simulink model "NMPCLib"  (R2018a)
settings: Solver=VariableStepAuto  StartTime=0.0  StopTime=4000  RelTol=1e-3  EnableMultiTasking=on
values from neighbouring files (symbols this model uses):
  Cai = 3.3*0.001    (= 0.0033)    [Data.m]
  Cair = 0.3    [Data.m]    (also in go.m = 0.4; go_params.m = 0.4)
  Cap = 45*3600    (= 162000)    [Data.m]
  Cb = 14000*3.56    (= 49840)    [Data.m]
  Cc = 43667.5*0.896    (= 39126.08)    [Data.m]
  Cd = 0.4*0.996    (= 0.3984)    [Data.m]
  Ci = 5*0.001    (= 0.005)    [Data.m]
  Cl = 560*0.896    (= 501.76)    [Data.m]
  Co = 3000*0.921    (= 2763)    [Data.m]
  dU0 = 0*ones(Usize,1)    [go.m]
  g = 9.8    [Data.m]    (also in go.m; go_params.m)
  Ja = 0.7282    [Data.m]
  Jb = 0.7282    [Data.m]
  Kb = 9.6    [Data.m]
  Kre_a = 0.10    (= 0.1)    [Data.m]
  Kre_b = 0.12    [Data.m]
  Ktr = 4.4    [Data.m]
  M = 288    [Data.m]    (also in go.m; go_params.m)
  Miur0 = 0.01    [Data.m]    (also in go.m; go_params.m)
  Np = ceil(45/6.650)    [Data.m]
  Ns = ceil(72/12.6)    [Data.m]
  pair = 1.25    [Data.m]    (also in go.m = 0.9643; go_params.m = 0.9643)
  Qrd = as*(GD*cos(ang)+Gd)    [Data.m]
  Raic = 1/(Aaic*h_air)    (= 406.940119575)    [Data.m]
  Rail = 1/(Alai*h_air)    (= 951.594301092)    [Data.m]
  Rba = 1/(Aba*k_litio)    (= 0.0922236978014)    [Data.m]
  Rbi = 1/(Abi*k_litio)    (= 0.0277596414787)    [Data.m]
  Rbo = 1/(Abo*k_litio)    (= 0.0277596414787)    [Data.m]
  Rca = 1/(Aca*k_alum)    (= 0.0351745602272)    [Data.m]
  Rcai = 1/(Aaic*k_alum)    (= 0.0505515676491)    [Data.m]
  Rdl = 1/(Adl*(k_alum*km_Crem))    (= 0.0199076286033)    [Data.m]
  Rib = 1/(Abi*h_air)    (= 321.584769745)    [Data.m]
  Rio = 1/(Aio*h_air)    (= 898.634076204)    [Data.m]
  Rlai = 1/(Alai*k_alum)    (= 0.118210472185)    [Data.m]
  Rlc = 1/(Alc*k_alum)    (= 0.115635579282)    [Data.m]
  Roa = 1/(Aoa*k_alum)    (= 0.029420140793)    [Data.m]
  Rob = 1/(Abo*k_alum)    (= 0.0399484186019)    [Data.m]
  Roi = 1/(Aio*k_alum)    (= 0.111631562261)    [Data.m]
  Rwr = 0.3302    [Data.m]    (also in go.m = 0.58; go_params.m = 0.58)
  Surf = 0.94243    [Data.m]    (also in go.m; go_params.m)
  Tai0 = 25    [Data.m]
  Tb0 = 25    [Data.m]
  Tc0 = 25    [Data.m]
  Td0 = 25    [Data.m]
  Ti0 = 25    [Data.m]
  Tl0 = 25    [Data.m]
  To0 = 25    [Data.m]
  U0 = 0*ones(Usize,1)    [go.m]
  Udc = 72    [Data.m]
libraries: simulink x6
settings Model: Creator=stajeddi  LastModifiedBy=yesid
settings DataIOCC: LimitDataPoints=on
settings OptimizationCC: LifeSpan=inf
settings DebuggingCC: AllowSymbolicDim=off  SFUnexpectedBacktrackingDiag=warning  SFNoUnconditionalDefaultTransitionDiag=warning  SFExecutionAtInitializationDiag=none
settings ModelReferenceCC: PropagateSignalLabelsOutOfModel=off
settings CodeAppCC: StateflowObjectComments=on
settings GRTTargetCC: TargetLangStandard=C89/C90 (ANSI)
settings ConfigComp: CovMetricSettings=dw  CovHtmlReporting=on  CovSaveCumulativeToWorkspaceVar=on  CovSaveSingleToWorkspaceVar=on  CovExternalEMLEnable=off

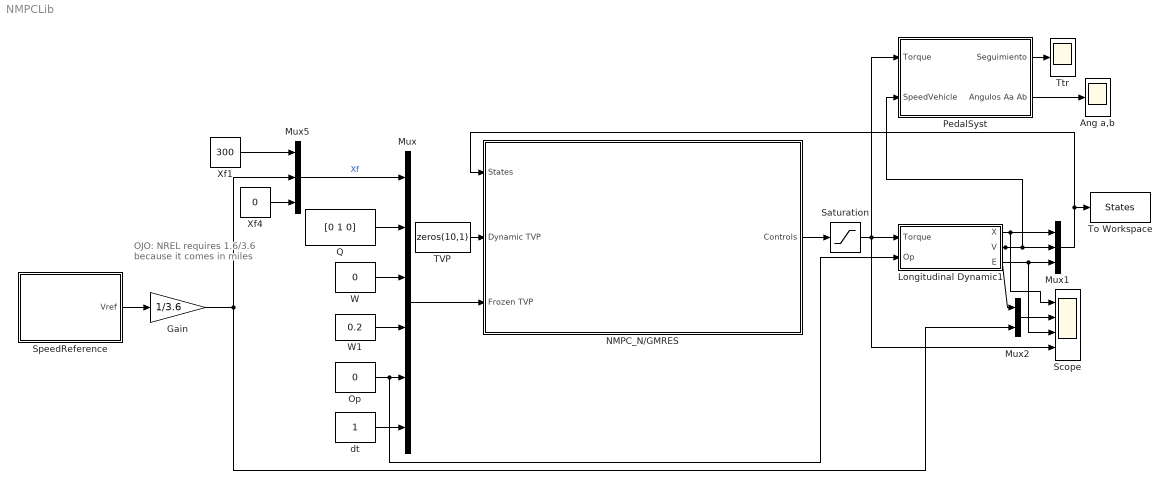
== system NMPCLib ==
  note: OJO: NREL requires
      | 1.6/3.6 because it
      | comes in miles
  Ang a,b : Scope
  Gain : Gain  Gain=1/3.6
  Longitudinal Dynamic1 : Subsystem
  Mux : Mux  Inputs=6
  Mux1 : Mux  Inputs=3
  Mux2 : Mux  Inputs=2
  Mux5 : Mux  Inputs=3
  NMPC_N/GMRES : Subsystem
  Op : Constant  Value=0
  PedalSyst : Subsystem
  Q : Constant  Value=[0 1 0]
  Saturation : Saturate  UpperLimit=220  LowerLimit=-220
  Scope : Scope  NumInputPorts=4
  "SpeedReference " : Subsystem
  TVP : Constant  Value=zeros(10,1)
  To Workspace : ToWorkspace  VariableName=States  SaveFormat=Timeseries  SampleTime=-1
  "Ttr " : Scope
  W : Constant  Value=0
  W1 : Constant  Value=0.2
  Xf1 : Constant  Value=300
  Xf4 : Constant  Value=0
  dt : Constant
  wires:
  Mux/1 -> NMPC_N/GMRES/3(Frozen TVP)
  Q/1 -> Mux/2
  W/1 -> Mux/3
  Mux5/1 -> Mux/1  "Xf"
  TVP/1 -> NMPC_N/GMRES/2(Dynamic TVP)
  Longitudinal Dynamic1/1(X) -> Scope/1, Mux1/1
  Longitudinal Dynamic1/2(V) -> Mux2/1, PedalSyst/2(SpeedVehicle), Mux1/2
  Xf1/1 -> Mux5/1
  Op/1 -> Longitudinal Dynamic1/2("Op "), Mux/5
  Mux2/1 -> Scope/2
  W1/1 -> Mux/4
  dt/1 -> Mux/6
  Xf4/1 -> Mux5/3
  Longitudinal Dynamic1/3(E) -> Scope/3, Mux1/3
  "SpeedReference "/1(Vref) -> Gain/1
  PedalSyst/1(Seguimiento) -> "Ttr "/1
  PedalSyst/2(Angulos Aa Ab) -> Ang a,b/1
  NMPC_N/GMRES/1(Controls) -> Saturation/1
  Saturation/1 -> PedalSyst/1(Torque), Scope/4, Longitudinal Dynamic1/1(Torque)
  Gain/1 -> Mux2/2, Mux5/2
  Mux1/1 -> To Workspace/1, NMPC_N/GMRES/1(States)

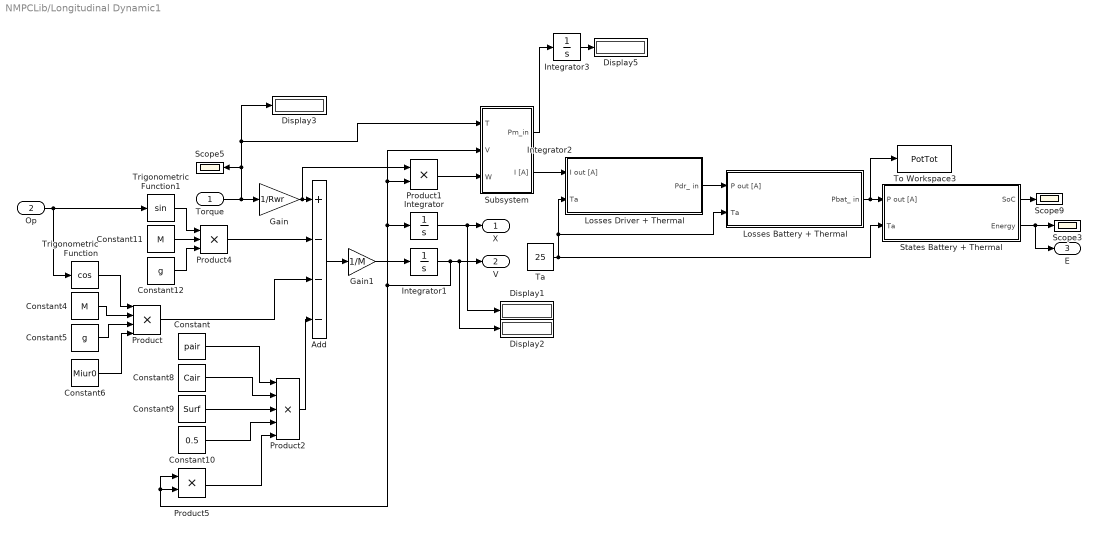
== system NMPCLib/Longitudinal Dynamic1 ==
  Torque : Inport
  "Op " : Inport  Port=2
  Add : Sum  Inputs=+---
  Constant : Constant  Value=pair
  Constant10 : Constant  Value=0.5
  Constant11 : Constant  Value=M
  Constant12 : Constant  Value=g
  Constant4 : Constant  Value=M
  Constant5 : Constant  Value=g
  Constant6 : Constant  Value=Miur0
  Constant8 : Constant  Value=Cair
  Constant9 : Constant  Value=Surf
  Display{1..3,5} (4 alike) : Display
  Gain : Gain  Gain=1/Rwr
  Gain1 : Gain  Gain=1/M
  Integrator{,1..3} (4 alike) : Integrator
  Losses Battery + Thermal : Subsystem
  Losses Driver + Thermal : Subsystem
  Product : Product  Inputs=4
  Product1 : Product
  Product2 : Product  Inputs=5
  Product4 : Product  Inputs=3
  Product5 : Product
  Scope3 : Scope
  Scope5 : Scope
  Scope9 : Scope
  States Battery + Thermal : Subsystem
  Subsystem : Subsystem
  Ta : Constant  Value=25
  To Workspace3 : ToWorkspace  VariableName=PotTot  SaveFormat=Timeseries  SampleTime=-1
  Trigonometric Function : Trigonometry  Operator=cos
  Trigonometric Function1 : Trigonometry
  X : Outport
  V : Outport  Port=2
  E : Outport  Port=3
  wires:
  Integrator/1 -> X/1, Display1/1
  Product2/1 -> Add/4
  Product5/1 -> Product2/5
  Constant10/1 -> Product2/4
  Constant8/1 -> Product2/2
  Constant/1 -> Product2/1
  Constant9/1 -> Product2/3
  Product/1 -> Add/3
  Constant6/1 -> Product/4
  Trigonometric Function/1 -> Product/1
  Constant5/1 -> Product/3
  Constant4/1 -> Product/2
  Add/1 -> Gain1/1
  "Op "/1 -> Trigonometric Function1/1, Trigonometric Function/1
  Product4/1 -> Add/2
  Gain/1 -> Product1/1, Add/1
  Constant12/1 -> Product4/3
  Trigonometric Function1/1 -> Product4/1
  Constant11/1 -> Product4/2
  Gain1/1 -> Integrator1/1
  Integrator1/1 -> V/1, Display2/1, Product1/2, Subsystem/2(V), Integrator/1, Product5/1, Product5/2
  Product1/1 -> Subsystem/3(W)
  Subsystem/1("Pm_in ") -> Integrator3/1
  Integrator3/1 -> Display5/1
  Subsystem/2(I [A]) -> Losses Driver + Thermal/1(I out [A])
  Losses Battery + Thermal/1(Pbat_ in) -> To Workspace3/1, States Battery + Thermal/1(P out [A])
  Ta/1 -> States Battery + Thermal/2(Ta), Losses Battery + Thermal/2(Ta), Losses Driver + Thermal/2(Ta)
  States Battery + Thermal/1(SoC) -> Scope9/1
  States Battery + Thermal/2(Energy) -> E/1, Scope3/1
  Torque/1 -> Gain/1, Scope5/1, Subsystem/1(T), Display3/1
  Losses Driver + Thermal/1(Pdr_ in) -> Losses Battery + Thermal/1(P out [A])

== system NMPCLib/NMPC_N//GMRES ==
  States : Inport
  Dynamic TVP : Inport  Port=2
  Frozen TVP : Inport  Port=3
  Solver : MATLAB Function  TreatAsAtomicUnit=on
  U0 : UnitDelay  InitialCondition=U0  SampleTime=-1
  dU0 : UnitDelay  InitialCondition=dU0  SampleTime=-1
  Controls : Outport
  wires:
  States/1 -> Solver/3(x0)
  Frozen TVP/1 -> Solver/5(TVP_f)
  Solver/3(Control) -> Controls/1
  Solver/2(U) -> U0/1
  U0/1 -> Solver/2(U0)
  Solver/1(dU) -> dU0/1
  dU0/1 -> Solver/1(dU0)
  Dynamic TVP/1 -> Solver/4(TVP)

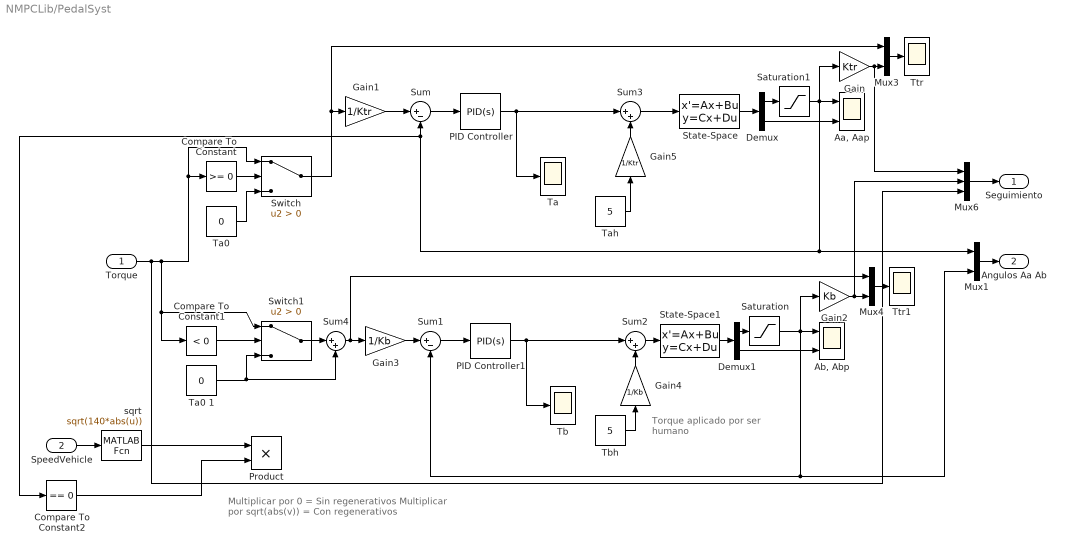
== system NMPCLib/PedalSyst ==
  note: Torque aplicado
      | por ser humano
  note: Multiplicar por 0                 = Sin regenerativos
      | Multiplicar por sqrt(abs(v)) = Con regenerativos
  Torque : Inport
  SpeedVehicle : Inport  Port=2
  "Aa, Aap" : Scope  NumInputPorts=2
  "Ab, Abp" : Scope  NumInputPorts=2
  Compare To Constant : simulink/Logic and Bit Operations/Compare To Constant  relop=>=  const=0  OutDataTypeStr=boolean
  Compare To Constant1 : simulink/Logic and Bit Operations/Compare To Constant  relop=<  const=0  OutDataTypeStr=boolean
  Compare To Constant2 : simulink/Logic and Bit Operations/Compare To Constant  relop===  const=0  OutDataTypeStr=boolean
  Demux : Demux  Outputs=2
  Demux1 : Demux  Outputs=2
  Gain : Gain  Gain=Ktr
  Gain1 : Gain  Gain=1/Ktr
  Gain2 : Gain  Gain=Kb
  Gain3 : Gain  Gain=1/Kb
  Gain4 : Gain  Gain=1/Kb
  Gain5 : Gain  Gain=1/Ktr
  Mux1 : Mux  Inputs=2
  Mux3 : Mux  Inputs=2
  Mux4 : Mux  Inputs=2
  Mux6 : Mux  Inputs=3
  PID Controller : simulink/Continuous/PID Controller  Controller=PID  TimeDomain=Continuous-time  SampleTime=-1  IntegratorMethod=Forward Euler  FilterMethod=Forward Euler  Form=Parallel  UseFilter=on  ControllerParametersSource=internal  P=1.77054619183816  I=0.294850673068489  D=2.09654617749741  N=11.2597730875944  InitialConditionSource=internal  InitialConditionForIntegrator=0  InitialConditionForFilter=0  ExternalReset=none  LimitOutput=off  UpperSaturationLimit=inf  LowerSaturationLimit=-inf  LinearizeAsGain=on  AntiWindupMode=none  Kb=1  TrackingMode=off  Kt=1  PParamMin=[]  PParamMax=[]  IParamMin=[]  IParamMax=[]  DParamMin=[]  DParamMax=[]  NParamMin=[]  NParamMax=[]  KbParamMin=[]  KbParamMax=[]  KtParamMin=[]  KtParamMax=[]  POutMin=[]  POutMax=[]  IOutMin=[]  IOutMax=[]  DOutMin=[]  DOutMax=[]  NOutMin=[]  NOutMax=[]  KbOutMin=[]  KbOutMax=[]  KtOutMin=[]  KtOutMax=[]  IntegratorOutMin=[]  IntegratorOutMax=[]  FilterOutMin=[]  FilterOutMax=[]  SumOutMin=[]  SumOutMax=[]  SumI1OutMin=[]  SumI1OutMax=[]  SumI2OutMin=[]  SumI2OutMax=[]  SumI3OutMin=[]  SumI3OutMax=[]  SumDOutMin=[]  SumDOutMax=[]  SaturationOutMin=[]  SaturationOutMax=[]  IntegratorContinuousStateAttributes=''  IntegratorStateMustResolveToSignalObject=off  IntegratorRTWStateStorageClass=Auto  FilterContinuousStateAttributes=''  FilterStateMustResolveToSignalObject=off  FilterRTWStateStorageClass=Auto  DifferentiatorICPrevScaledInput=0  DifferentiatorOutMin=[]  DifferentiatorOutMax=[]  FilterDiffOutCoefMin=[]  FilterDiffOutCoefMax=[]  SumDenOutMin=[]  SumDenOutMax=[]  SumNumOutMin=[]  SumNumOutMax=[]  ReciprocalOutMin=[]  ReciprocalOutMax=[]  DivideOutMin=[]  DivideOutMax=[]  TunerSelectOption=Transfer Function Based (PID Tuner App)
  PID Controller1 : simulink/Continuous/PID Controller  Controller=PID  TimeDomain=Continuous-time  SampleTime=-1  IntegratorMethod=Forward Euler  FilterMethod=Forward Euler  Form=Parallel  UseFilter=on  ControllerParametersSource=internal  P=1.6606981855622  I=0.298062139202914  D=2.01708670293522  N=30.9007600848216  InitialConditionSource=internal  InitialConditionForIntegrator=0  InitialConditionForFilter=0  ExternalReset=none  LimitOutput=off  UpperSaturationLimit=inf  LowerSaturationLimit=-inf  LinearizeAsGain=on  AntiWindupMode=none  Kb=1  TrackingMode=off  Kt=1  PParamMin=[]  PParamMax=[]  IParamMin=[]  IParamMax=[]  DParamMin=[]  DParamMax=[]  NParamMin=[]  NParamMax=[]  KbParamMin=[]  KbParamMax=[]  KtParamMin=[]  KtParamMax=[]  POutMin=[]  POutMax=[]  IOutMin=[]  IOutMax=[]  DOutMin=[]  DOutMax=[]  NOutMin=[]  NOutMax=[]  KbOutMin=[]  KbOutMax=[]  KtOutMin=[]  KtOutMax=[]  IntegratorOutMin=[]  IntegratorOutMax=[]  FilterOutMin=[]  FilterOutMax=[]  SumOutMin=[]  SumOutMax=[]  SumI1OutMin=[]  SumI1OutMax=[]  SumI2OutMin=[]  SumI2OutMax=[]  SumI3OutMin=[]  SumI3OutMax=[]  SumDOutMin=[]  SumDOutMax=[]  SaturationOutMin=[]  SaturationOutMax=[]  IntegratorContinuousStateAttributes=''  IntegratorStateMustResolveToSignalObject=off  IntegratorRTWStateStorageClass=Auto  FilterContinuousStateAttributes=''  FilterStateMustResolveToSignalObject=off  FilterRTWStateStorageClass=Auto  DifferentiatorICPrevScaledInput=0  DifferentiatorOutMin=[]  DifferentiatorOutMax=[]  FilterDiffOutCoefMin=[]  FilterDiffOutCoefMax=[]  SumDenOutMin=[]  SumDenOutMax=[]  SumNumOutMin=[]  SumNumOutMax=[]  ReciprocalOutMin=[]  ReciprocalOutMax=[]  DivideOutMin=[]  DivideOutMax=[]  TunerSelectOption=Transfer Function Based (PID Tuner App)
  Product : Product
  Saturation : Saturate  UpperLimit=0  LowerLimit=-50
  Saturation1 : Saturate  UpperLimit=50  LowerLimit=0
  State-Space : StateSpace  A=[0 1; -Kre_a/Ja 0]  B=[0; 1/Ja]  C=[1 0; 0 1]  D=[0; 0]  InitialCondition=[0 0]
  State-Space1 : StateSpace  A=[0 1; -Kre_b/Jb 0]  B=[0; 1/Jb]  C=[1 0; 0 1]  D=[0; 0]  InitialCondition=[0 0]
  Sum : Sum  Inputs=|+-
  Sum1 : Sum  Inputs=|+-
  Sum2 : Sum  Inputs=|++
  Sum3 : Sum  Inputs=|++
  Sum4 : Sum  Inputs=|++
  Switch : Switch  Criteria=u2 > Threshold
  Switch1 : Switch  Criteria=u2 > Threshold
  Ta : Scope
  "Ta0 " : Constant  Value=0
  Ta0 1 : Constant  Value=0
  Tah : Constant  Value=5
  Tb : Scope
  "Tbh " : Constant  Value=5
  Ttr : Scope
  Ttr1 : Scope
  sqrt : MATLABFcn  MATLABFcn=sqrt(140*abs(u))
  Seguimiento : Outport
  Angulos Aa Ab : Outport  Port=2
  wires:
  "Ta0 "/1 -> Switch/3
  Gain2/1 -> Mux6/2, Mux4/2
  Gain5/1 -> Sum3/2
  Torque/1 -> Switch/1, Compare To Constant/1, Switch1/1, Compare To Constant1/1, Mux6/3
  PID Controller1/1 -> Sum2/1, Tb/1
  Switch/1 -> Mux3/1, Gain1/1
  Gain/1 -> Mux6/1, Mux3/2
  Gain1/1 -> Sum/1
  Ta0 1/1 -> Sum4/2, Switch1/3
  Tah/1 -> Gain5/1
  Compare To Constant/1 -> Switch/2
  PID Controller/1 -> Sum3/1, Ta/1
  Sum/1 -> PID Controller/1
  Sum3/1 -> State-Space/1
  State-Space/1 -> Demux/1
  Compare To Constant1/1 -> Switch1/2
  Mux6/1 -> Seguimiento/1
  Mux4/1 -> Ttr1/1
  Sum2/1 -> State-Space1/1
  Demux/2 -> "Aa, Aap"/2
  "Tbh "/1 -> Gain4/1
  State-Space1/1 -> Demux1/1
  Mux3/1 -> Ttr/1
  Sum1/1 -> PID Controller1/1
  Gain4/1 -> Sum2/2
  Gain3/1 -> Sum1/1
  Demux1/2 -> "Ab, Abp"/2
  Mux1/1 -> Angulos Aa Ab/1
  Demux1/1 -> Saturation/1
  Saturation/1 -> Mux1/2, Sum1/2, Gain2/1, "Ab, Abp"/1
  Demux/1 -> Saturation1/1
  Saturation1/1 -> Sum/2, Compare To Constant2/1, Mux1/1, Gain/1, "Aa, Aap"/1
  Switch1/1 -> Sum4/1
  Sum4/1 -> Mux4/1, Gain3/1
  SpeedVehicle/1 -> sqrt/1
  sqrt/1 -> Product/1
  Compare To Constant2/1 -> Product/2

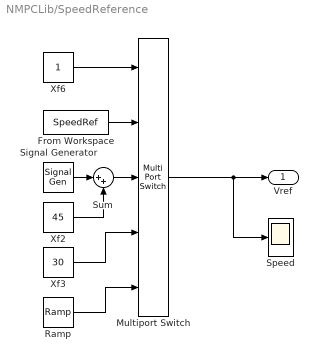
== system NMPCLib/SpeedReference  ==
  From Workspace : FromWorkspace  VariableName=SpeedRef  SampleTime=0
  Multiport Switch : MultiPortSwitch  Inputs=4
  Ramp : simulink/Sources/Ramp  slope=0.03  start=0  InitialOutput=0
  Signal Generator : SignalGenerator  Units=rad/sec
  "Speed " : Scope
  Sum : Sum  Inputs=|++
  Xf2 : Constant  Value=45
  Xf3 : Constant  Value=30
  Xf6 : Constant
  Vref : Outport
  wires:
  Signal Generator/1 -> Sum/1
  From Workspace/1 -> Multiport Switch/2
  Xf6/1 -> Multiport Switch/1
  Ramp/1 -> Multiport Switch/5
  Xf3/1 -> Multiport Switch/4
  Xf2/1 -> Sum/2
  Sum/1 -> Multiport Switch/3
  Multiport Switch/1 -> "Speed "/1, Vref/1

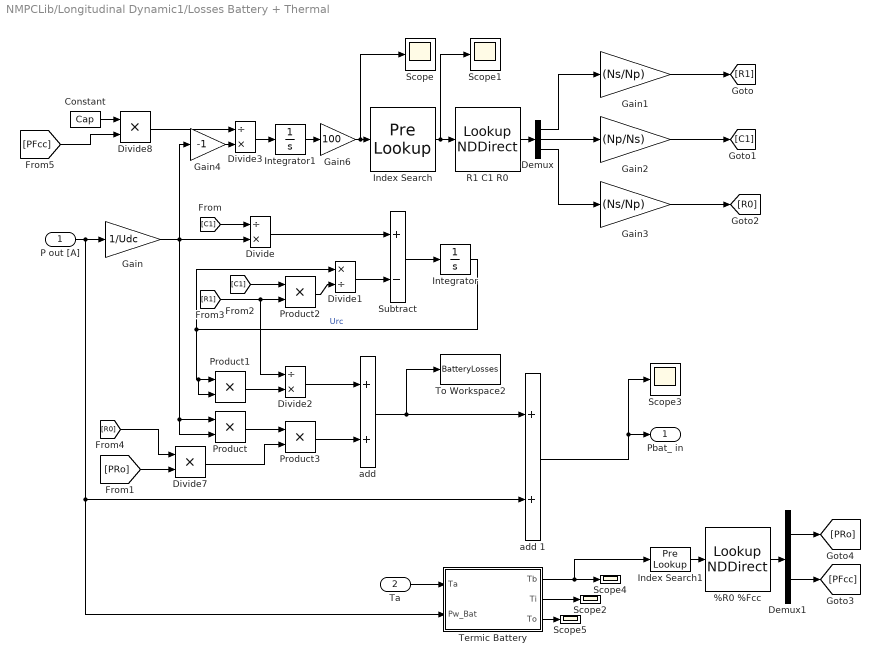
== system NMPCLib/Longitudinal Dynamic1/Losses Battery + Thermal ==
  P out [A] : Inport
  Ta : Inport  Port=2
  "%R0 %Fcc " : LookupNDDirect  InputsSelectThisObjectFromTable=Vector  Table=|
      | [7.33  0.71;
      | 4.97  0.75;
      | 3.58  0.78;
      | 2.69  0.82;
      | 2.07  0.86;
      | 1.63  0.89;
      | 1.30  0.93;
      | 1.14  0.97;
      | 1.00  1.00;
      | 0.91  1.04;
      | 0.84  1.07;
      | 0.77  1.09;]'
  Constant : Constant  Value=Cap
  Demux : Demux  Outputs=3
  Demux1 : Demux  Outputs=2
  Divide : Product  Inputs=/*
  Divide1 : Product  Inputs=*/
  Divide2 : Product  Inputs=/*
  Divide3 : Product  Inputs=/*
  Divide7 : Product  Inputs=**
  Divide8 : Product  Inputs=**
  Gain : Gain  Gain=1/Udc
  Gain1 : Gain  Gain=(Ns/Np)
  Gain2 : Gain  Gain=(Np/Ns)
  Gain3 : Gain  Gain=(Ns/Np)
  Gain4 : Gain  Gain=-1
  Gain6 : Gain  Gain=100
  Index Search : PreLookup  BreakpointsData=|  OutputSelection=Index only
      | [2.273
      | 4.545
      | 6.818
      | 9.091
      | 11.364
      | 13.636
      | 15.909
      | 18.182
      | 20.455
      | 22.727
      | 25.000
      | 27.273
      | 29.545
      | 31.818
      | 34.091
      | 36.364
      | 38.636
      | 40.909
      | 43.182
      | 45.455
      | 47.727
      | 50.000
      | 52.273
      | 54.545
      | 56.818
      | 59.091
      | 61.364
      | 63.636
      | 65.909
      | 68.182
      | 70.455
      | 72.727
      | 75.000
      | 77.273
      | 79.545
      | 81.818
      | 84.091
      | 86.364
      | 88.636
      | 90.909
      | 93.182
      | 95.455
      | 97.727
      | 100.000]
  Index Search1 : PreLookup  BreakpointsData="[-15 -10 -5 0  5 10  15 20 25 30 35 40]"  OutputSelection=Index only
  Integrator : Integrator
  Integrator1 : Integrator  InitialCondition=1
  Product{,1..3} (4 alike) : Product
  "R1 C1 R0 " : LookupNDDirect  InputsSelectThisObjectFromTable=Vector  Table=|
      | [0.046  1443.329 0.260;
      | 0.163	383.931	0.260;
      | 0.264	202.535	0.262;
      | 0.301	109.504	0.263;
      | 0.303	99.992	0.260;
      | 0.303	107.088	0.263;
      | 0.298	126.400	0.262;
      | 0.307	131.885	0.263;
      | 0.303	119.317	0.260;
      | 0.304	125.895	0.260;
      | 0.309	113.359	0.260;
      | 0.307	107.787	0.260;
      | 0.306	117.780	0.262;
      | 0.313	104.457	0.262;
      | 0.310	100.585	0.258;
      | 0.304	136.742	0.260;
      | 0.310	126.376	0.262;
      | 0.313	126.403	0.260;
      | 0.309	110.120	0.257;
      | 0.315	114.389	0.258;
      | 0.314	98.257	0.260;
      | 0.314	95.395	0.260;
      | 0.319	88.712	0.257;
      | 0.320	77.705	0.258;
      | 0.319	78.111	0.258;
      | 0.325	69.286	0.260;
      | 0.322	90.719	0.257;
      | 0.331	91.019	0.262;
      | 0.313	100.060	0.257;
      | 0.317	108.165	0.262;
      | 0.313	130.331	0.258;
      | 0.304	128.624	0.255;
      | 0.300	139.477	0.253;
      | 0.303	143.003	0.255;
      | 0.313	129.373	0.258;
      | 0.318	129.417	0.258;
      | 0.313	107.012	0.255;
      | 0.326	96.506	0.260;
      | 0.328	83.578	0.258;
      | 0.337	95.942	0.263;
      | 0.344	86.032	0.267;
      | 0.351	59.468	0.270;
      | 0.318	101.474	0.255;
      | 0.283	133.248	0.127;]'
  Scope{,1..5} (6 alike) : Scope
  Subtract : Sum  Inputs=+-
  "Termic Battery " : Subsystem
  To Workspace2 : ToWorkspace  VariableName=BatteryLosses  SaveFormat=Timeseries  SampleTime=-1
  "add " : Sum
  add 1 : Sum
  Pbat_ in : Outport
  wires:
  P out [A]/1 -> "Termic Battery "/2(Pw_Bat), add 1/2, Gain/1
  Gain/1 -> Gain4/1, Divide/2, Product/2, Product/1
  Divide/1 -> Subtract/1
  Divide1/1 -> Subtract/2
  Subtract/1 -> Integrator/1
  Integrator/1 -> Divide1/1, Product1/2, Product1/1  "Urc"
  add 1/1 -> Scope3/1, Pbat_ in/1
  Divide3/1 -> Integrator1/1
  Index Search/1 -> Scope1/1, "R1 C1 R0 "/1
  "R1 C1 R0 "/1 -> Demux/1
  Integrator1/1 -> Gain6/1
  Gain6/1 -> Scope/1, Index Search/1
  Demux/3 -> Gain3/1
  Demux/2 -> Gain2/1
  Demux/1 -> Gain1/1
  [C1] -> Divide/1
  Product2/1 -> Divide1/2
  [R1] -> Divide2/1, Product2/2
  [C1] -> Product2/1
  Product1/1 -> Divide2/2
  Divide2/1 -> "add "/1
  Product/1 -> Product3/1
  Product3/1 -> "add "/2
  "add "/1 -> add 1/1, To Workspace2/1
  Gain1/1 -> [R1]
  Gain2/1 -> [C1]
  Gain3/1 -> [R0]
  Ta/1 -> "Termic Battery "/1(Ta)
  "Termic Battery "/3(To) -> Scope5/1
  "Termic Battery "/2(Ti) -> Scope2/1
  Index Search1/1 -> "%R0 %Fcc "/1
  "Termic Battery "/1(Tb) -> Index Search1/1, Scope4/1
  "%R0 %Fcc "/1 -> Demux1/1
  Demux1/2 -> [PFcc]
  Demux1/1 -> [PRo]
  [PRo] -> Divide7/2
  Divide7/1 -> Product3/2
  [R0] -> Divide7/1
  Gain4/1 -> Divide3/2
  Divide8/1 -> Divide3/1
  Constant/1 -> Divide8/1
  [PFcc] -> Divide8/2

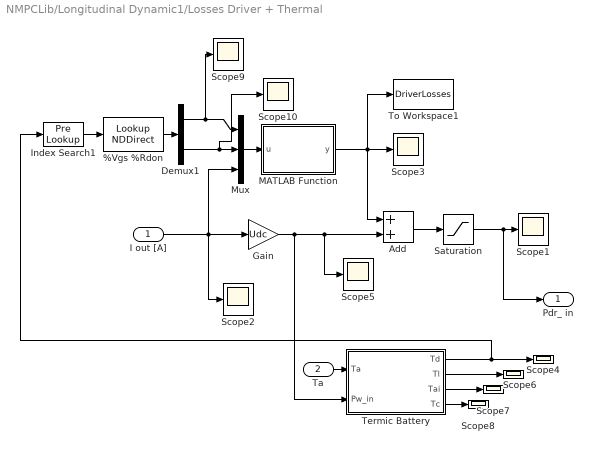
== system NMPCLib/Longitudinal Dynamic1/Losses Driver + Thermal ==
  I out [A] : Inport
  Ta : Inport  Port=2
  "%Vgs %Rdon " : LookupNDDirect  InputsSelectThisObjectFromTable=Vector  Table=|
      | [0.80   1.4;
      | 0.82   1.4;
      | 0.85   1.3;
      | 0.87   1.3;
      | 0.90   1.2;
      | 0.92   1.2;
      | 0.95   1.1;
      | 0.97   1.1;
      | 1.00   1.0;
      | 1.05   0.99;
      | 1.08   0.99;
      | 1.11   0.98;
      | 1.13   0.98;
      | 1.15   0.97;
      | 1.20   0.97;
      | 1.22   0.96;
      | 1.25   0.95;
      | 1.27   0.94;
      | 1.30   0.93;
      | 1.35   0.92;
      | 1.40   0.91;
      | 1.45   0.90;
      | 1.50   0.89;
      | 1.55   0.88;
      | 1.60   0.87;
      | 1.65   0.86;
      | 1.70   0.85;
      | 1.75   0.84;
      | 1.80   0.83;
      | 1.85   0.81;
      | 1.90   0.79;
      | 1.95   0.78;
      | 2.00   0.77;
      | 2.05   0.76;
      | 2.10   0.74;]'
  Add : Sum
  Demux1 : Demux  Outputs=2
  Gain : Gain  Gain=Udc
  Index Search1 : PreLookup  BreakpointsData=[-15:5:155]  OutputSelection=Index only
  MATLAB Function : MATLAB Function  TreatAsAtomicUnit=on
  Mux : Mux  Inputs=3
  Saturation : Saturate  UpperLimit=4000  LowerLimit=-5000
  Scope{1..10} (10 alike) : Scope
  "Termic Battery " : Subsystem
  To Workspace1 : ToWorkspace  VariableName=DriverLosses  SaveFormat=Timeseries  SampleTime=-1
  Pdr_ in : Outport
  wires:
  I out [A]/1 -> Mux/3, Scope2/1, Gain/1
  Add/1 -> Saturation/1
  MATLAB Function/1(y) -> To Workspace1/1, Add/1, Scope3/1
  Saturation/1 -> Scope1/1, Pdr_ in/1
  "%Vgs %Rdon "/1 -> Demux1/1
  Index Search1/1 -> "%Vgs %Rdon "/1
  Demux1/1 -> Scope9/1, Mux/1
  Demux1/2 -> Scope10/1, Mux/2
  Ta/1 -> "Termic Battery "/1(Ta)
  Gain/1 -> "Termic Battery "/2(Pw_in), Add/2, Scope5/1
  "Termic Battery "/4(Tc) -> Scope8/1
  "Termic Battery "/3(Tai) -> Scope7/1
  "Termic Battery "/2(Tl) -> Scope6/1
  "Termic Battery "/1(Td) -> Index Search1/1, Scope4/1
  Mux/1 -> MATLAB Function/1(u)

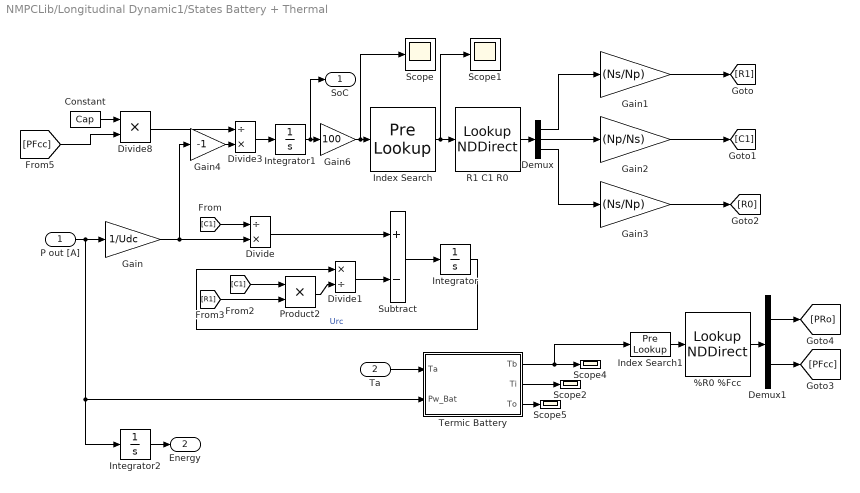
== system NMPCLib/Longitudinal Dynamic1/States Battery + Thermal ==
  P out [A] : Inport
  Ta : Inport  Port=2
  "%R0 %Fcc " : LookupNDDirect  InputsSelectThisObjectFromTable=Vector  Table=|
      | [7.33  0.71;
      | 4.97  0.75;
      | 3.58  0.78;
      | 2.69  0.82;
      | 2.07  0.86;
      | 1.63  0.89;
      | 1.30  0.93;
      | 1.14  0.97;
      | 1.00  1.00;
      | 0.91  1.04;
      | 0.84  1.07;
      | 0.77  1.09;]'
  Constant : Constant  Value=Cap
  Demux : Demux  Outputs=3
  Demux1 : Demux  Outputs=2
  Divide : Product  Inputs=/*
  Divide1 : Product  Inputs=*/
  Divide3 : Product  Inputs=/*
  Divide8 : Product  Inputs=**
  Gain : Gain  Gain=1/Udc
  Gain1 : Gain  Gain=(Ns/Np)
  Gain2 : Gain  Gain=(Np/Ns)
  Gain3 : Gain  Gain=(Ns/Np)
  Gain4 : Gain  Gain=-1
  Gain6 : Gain  Gain=100
  Index Search : PreLookup  BreakpointsData=|  OutputSelection=Index only
      | [2.273
      | 4.545
      | 6.818
      | 9.091
      | 11.364
      | 13.636
      | 15.909
      | 18.182
      | 20.455
      | 22.727
      | 25.000
      | 27.273
      | 29.545
      | 31.818
      | 34.091
      | 36.364
      | 38.636
      | 40.909
      | 43.182
      | 45.455
      | 47.727
      | 50.000
      | 52.273
      | 54.545
      | 56.818
      | 59.091
      | 61.364
      | 63.636
      | 65.909
      | 68.182
      | 70.455
      | 72.727
      | 75.000
      | 77.273
      | 79.545
      | 81.818
      | 84.091
      | 86.364
      | 88.636
      | 90.909
      | 93.182
      | 95.455
      | 97.727
      | 100.000]
  Index Search1 : PreLookup  BreakpointsData="[-15 -10 -5 0  5 10  15 20 25 30 35 40]"  OutputSelection=Index only
  Integrator : Integrator
  Integrator1 : Integrator  InitialCondition=1
  Integrator2 : Integrator
  Product2 : Product
  "R1 C1 R0 " : LookupNDDirect  InputsSelectThisObjectFromTable=Vector  Table=|
      | [0.046  1443.329 0.260;
      | 0.163	383.931	0.260;
      | 0.264	202.535	0.262;
      | 0.301	109.504	0.263;
      | 0.303	99.992	0.260;
      | 0.303	107.088	0.263;
      | 0.298	126.400	0.262;
      | 0.307	131.885	0.263;
      | 0.303	119.317	0.260;
      | 0.304	125.895	0.260;
      | 0.309	113.359	0.260;
      | 0.307	107.787	0.260;
      | 0.306	117.780	0.262;
      | 0.313	104.457	0.262;
      | 0.310	100.585	0.258;
      | 0.304	136.742	0.260;
      | 0.310	126.376	0.262;
      | 0.313	126.403	0.260;
      | 0.309	110.120	0.257;
      | 0.315	114.389	0.258;
      | 0.314	98.257	0.260;
      | 0.314	95.395	0.260;
      | 0.319	88.712	0.257;
      | 0.320	77.705	0.258;
      | 0.319	78.111	0.258;
      | 0.325	69.286	0.260;
      | 0.322	90.719	0.257;
      | 0.331	91.019	0.262;
      | 0.313	100.060	0.257;
      | 0.317	108.165	0.262;
      | 0.313	130.331	0.258;
      | 0.304	128.624	0.255;
      | 0.300	139.477	0.253;
      | 0.303	143.003	0.255;
      | 0.313	129.373	0.258;
      | 0.318	129.417	0.258;
      | 0.313	107.012	0.255;
      | 0.326	96.506	0.260;
      | 0.328	83.578	0.258;
      | 0.337	95.942	0.263;
      | 0.344	86.032	0.267;
      | 0.351	59.468	0.270;
      | 0.318	101.474	0.255;
      | 0.283	133.248	0.127;]'
  Scope{,1..2,4..5} (5 alike) : Scope
  Subtract : Sum  Inputs=+-
  "Termic Battery " : Subsystem
  SoC : Outport
  Energy : Outport  Port=2
  wires:
  P out [A]/1 -> Integrator2/1, "Termic Battery "/2(Pw_Bat), Gain/1
  Gain/1 -> Gain4/1, Divide/2
  Divide/1 -> Subtract/1
  Divide1/1 -> Subtract/2
  Subtract/1 -> Integrator/1
  Integrator/1 -> Divide1/1  "Urc"
  Divide3/1 -> Integrator1/1
  Index Search/1 -> Scope1/1, "R1 C1 R0 "/1
  "R1 C1 R0 "/1 -> Demux/1
  Integrator1/1 -> SoC/1, Gain6/1
  Gain6/1 -> Scope/1, Index Search/1
  Demux/3 -> Gain3/1
  Demux/2 -> Gain2/1
  Demux/1 -> Gain1/1
  [C1] -> Divide/1
  Product2/1 -> Divide1/2
  [R1] -> Product2/2
  [C1] -> Product2/1
  Gain1/1 -> [R1]
  Gain2/1 -> [C1]
  Gain3/1 -> [R0]
  Ta/1 -> "Termic Battery "/1(Ta)
  "Termic Battery "/3(To) -> Scope5/1
  "Termic Battery "/2(Ti) -> Scope2/1
  Index Search1/1 -> "%R0 %Fcc "/1
  "Termic Battery "/1(Tb) -> Index Search1/1, Scope4/1
  "%R0 %Fcc "/1 -> Demux1/1
  Demux1/2 -> [PFcc]
  Demux1/1 -> [PRo]
  Gain4/1 -> Divide3/2
  Divide8/1 -> Divide3/1
  Constant/1 -> Divide8/1
  [PFcc] -> Divide8/2
  Integrator2/1 -> Energy/1

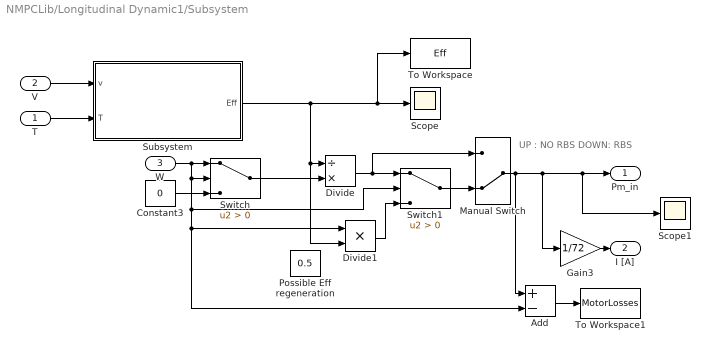
== system NMPCLib/Longitudinal Dynamic1/Subsystem ==
  note: UP      : NO RBS
      | DOWN: RBS
  T : Inport
  V : Inport  Port=2
  W : Inport  Port=3
  Add : Sum  Inputs=+-
  Constant3 : Constant  Value=0
  Divide : Product  Inputs=/*
  Divide1 : Product  Inputs=**
  Gain3 : Gain  Gain=1/72
  Manual Switch : ManualSwitch  CurrentSetting=0
  Possible Eff regeneration : Constant  Value=0.5
  Scope : Scope
  Scope1 : Scope
  Subsystem : Subsystem
  Switch : Switch  Criteria=u2 > Threshold
  Switch1 : Switch  Criteria=u2 > Threshold
  To Workspace : ToWorkspace  VariableName=Eff  SaveFormat=Timeseries  SampleTime=-1
  To Workspace1 : ToWorkspace  VariableName=MotorLosses  SaveFormat=Timeseries  SampleTime=-1
  "Pm_in " : Outport
  I [A] : Outport  Port=2
  wires:
  Gain3/1 -> I [A]/1
  W/1 -> Add/2, Divide1/1, Switch1/2, Switch/2, Switch/1
  Constant3/1 -> Switch/3
  Switch/1 -> Divide/2
  Divide/1 -> Manual Switch/1, Switch1/1
  Divide1/1 -> Switch1/3
  Switch1/1 -> Manual Switch/2
  Manual Switch/1 -> Add/1, Gain3/1, Scope1/1, "Pm_in "/1
  Subsystem/1(Eff) -> Divide1/2, Divide/1, To Workspace/1, Scope/1
  V/1 -> Subsystem/1(v)
  T/1 -> Subsystem/2(T)
  Add/1 -> To Workspace1/1

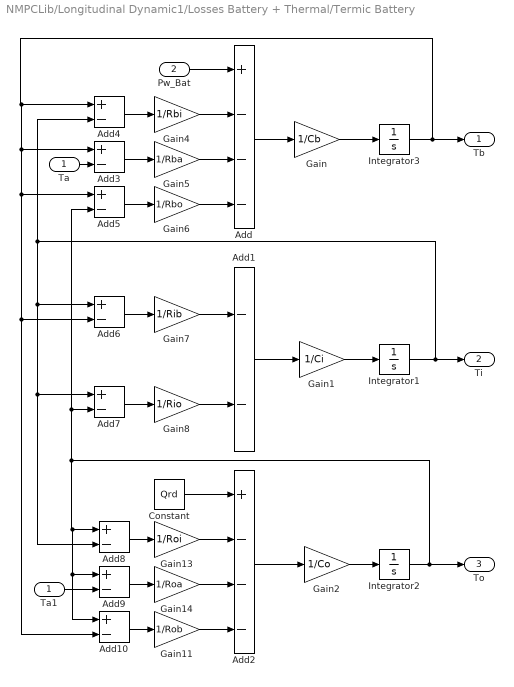
== system NMPCLib/Longitudinal Dynamic1/Losses Battery + Thermal/Termic Battery  ==
  Ta : Inport
  Pw_Bat : Inport  Port=2
  Add : Sum  Inputs=+---
  Add1 : Sum  Inputs=--
  Add{3..10} (8 alike) : Sum  Inputs=+-
  Add2 : Sum  Inputs=+---
  Constant : Constant  Value=Qrd
  Gain : Gain  Gain=1/Cb
  Gain1 : Gain  Gain=1/Ci
  Gain11 : Gain  Gain=1/Rob
  Gain13 : Gain  Gain=1/Roi
  Gain14 : Gain  Gain=1/Roa
  Gain2 : Gain  Gain=1/Co
  Gain4 : Gain  Gain=1/Rbi
  Gain5 : Gain  Gain=1/Rba
  Gain6 : Gain  Gain=1/Rbo
  Gain7 : Gain  Gain=1/Rib
  Gain8 : Gain  Gain=1/Rio
  Integrator1 : Integrator  InitialCondition=Ti0
  Integrator2 : Integrator  InitialCondition=To0
  Integrator3 : Integrator  InitialCondition=Tb0
  Ta1 : InportShadow
  Tb : Outport
  Ti : Outport  Port=2
  To : Outport  Port=3
  wires:
  Integrator3/1 -> Add3/1, Add5/1, Add10/2, Add6/2, Add4/1, Tb/1
  Integrator1/1 -> Add4/2, Add6/1, Add7/1, Add8/2, Ti/1
  Integrator2/1 -> Add7/2, Add5/2, Add10/1, Add9/1, Add8/1, To/1
  Add/1 -> Gain/1
  Add1/1 -> Gain1/1
  Add2/1 -> Gain2/1
  Gain/1 -> Integrator3/1
  Gain1/1 -> Integrator1/1
  Gain2/1 -> Integrator2/1
  Pw_Bat/1 -> Add/1
  Gain4/1 -> Add/2
  Gain5/1 -> Add/3
  Gain6/1 -> Add/4
  Gain7/1 -> Add1/1
  Gain8/1 -> Add1/2
  Constant/1 -> Add2/1
  Gain13/1 -> Add2/2
  Gain14/1 -> Add2/3
  Gain11/1 -> Add2/4
  Add4/1 -> Gain4/1
  Add6/1 -> Gain7/1
  Add8/1 -> Gain13/1
  Add9/1 -> Gain14/1
  Add10/1 -> Gain11/1
  Add7/1 -> Gain8/1
  Add5/1 -> Gain6/1
  Add3/1 -> Gain5/1
  Ta/1 -> Add3/2
  Ta1/1 -> Add9/2

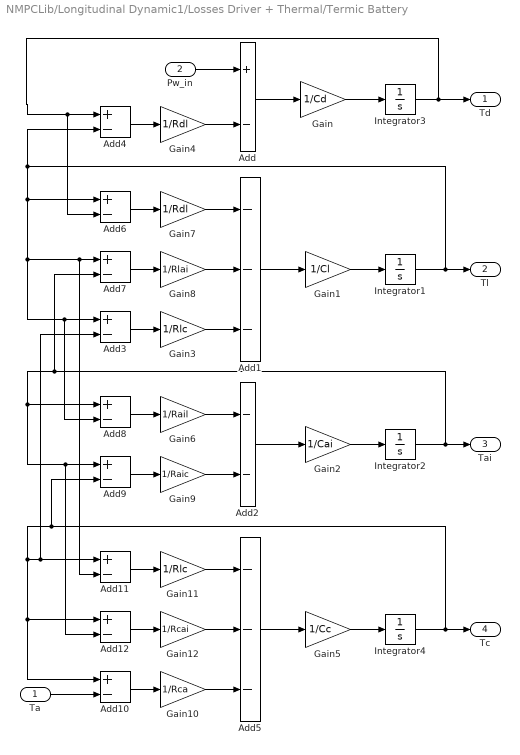
== system NMPCLib/Longitudinal Dynamic1/Losses Driver + Thermal/Termic Battery  ==
  Ta : Inport
  Pw_in : Inport  Port=2
  Add{,3..4,6..12} (10 alike) : Sum  Inputs=+-
  Add1 : Sum  Inputs=---
  Add2 : Sum  Inputs=--
  Add5 : Sum  Inputs=---
  Gain : Gain  Gain=1/Cd
  Gain1 : Gain  Gain=1/Cl
  Gain10 : Gain  Gain=1/Rca
  Gain11 : Gain  Gain=1/Rlc
  Gain12 : Gain  Gain=1/Rcai
  Gain2 : Gain  Gain=1/Cai
  Gain3 : Gain  Gain=1/Rlc
  Gain4 : Gain  Gain=1/Rdl
  Gain5 : Gain  Gain=1/Cc
  Gain6 : Gain  Gain=1/Rail
  Gain7 : Gain  Gain=1/Rdl
  Gain8 : Gain  Gain=1/Rlai
  Gain9 : Gain  Gain=1/Raic
  Integrator1 : Integrator  InitialCondition=Tl0
  Integrator2 : Integrator  InitialCondition=Tai0
  Integrator3 : Integrator  InitialCondition=Td0
  Integrator4 : Integrator  InitialCondition=Tc0
  Td : Outport
  Tl : Outport  Port=2
  Tai : Outport  Port=3
  Tc : Outport  Port=4
  wires:
  Integrator3/1 -> Add6/2, Add4/1, Td/1
  Integrator1/1 -> Add4/2, Add7/1, Add11/2, Add3/1, Add8/2, Add6/1, Tl/1
  Add/1 -> Gain/1
  Add1/1 -> Gain1/1
  Gain/1 -> Integrator3/1
  Gain1/1 -> Integrator1/1
  Pw_in/1 -> Add/1
  Gain4/1 -> Add/2
  Gain7/1 -> Add1/1
  Gain8/1 -> Add1/2
  Add4/1 -> Gain4/1
  Add6/1 -> Gain7/1
  Add7/1 -> Gain8/1
  Add3/1 -> Gain3/1
  Add9/1 -> Gain9/1
  Add8/1 -> Gain6/1
  Gain9/1 -> Add2/2
  Gain6/1 -> Add2/1
  Gain2/1 -> Integrator2/1
  Add2/1 -> Gain2/1
  Integrator2/1 -> Tai/1, Add7/2, Add8/1, Add9/1, Add12/2
  Add10/1 -> Gain10/1
  Add12/1 -> Gain12/1
  Add11/1 -> Gain11/1
  Gain12/1 -> Add5/2
  Gain11/1 -> Add5/1
  Gain5/1 -> Integrator4/1
  Add5/1 -> Gain5/1
  Integrator4/1 -> Tc/1, Add9/2, Add3/2, Add11/1, Add12/1, Add10/1
  Ta/1 -> Add10/2
  Gain3/1 -> Add1/3
  Gain10/1 -> Add5/3

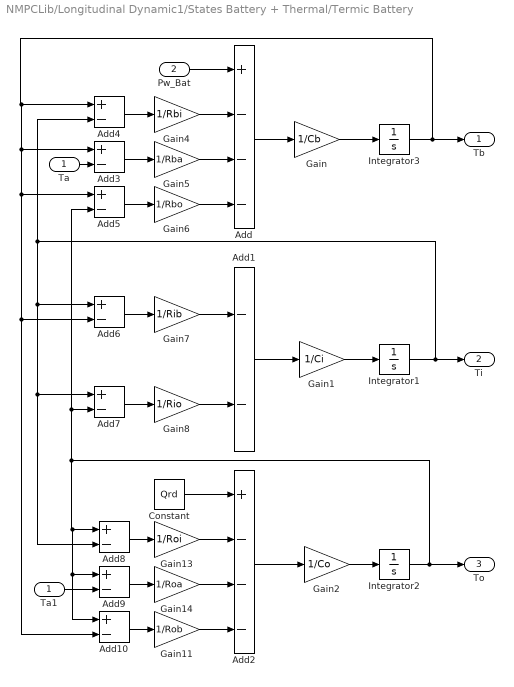
== system NMPCLib/Longitudinal Dynamic1/States Battery + Thermal/Termic Battery  ==
  Ta : Inport
  Pw_Bat : Inport  Port=2
  Add : Sum  Inputs=+---
  Add1 : Sum  Inputs=--
  Add{3..10} (8 alike) : Sum  Inputs=+-
  Add2 : Sum  Inputs=+---
  Constant : Constant  Value=Qrd
  Gain : Gain  Gain=1/Cb
  Gain1 : Gain  Gain=1/Ci
  Gain11 : Gain  Gain=1/Rob
  Gain13 : Gain  Gain=1/Roi
  Gain14 : Gain  Gain=1/Roa
  Gain2 : Gain  Gain=1/Co
  Gain4 : Gain  Gain=1/Rbi
  Gain5 : Gain  Gain=1/Rba
  Gain6 : Gain  Gain=1/Rbo
  Gain7 : Gain  Gain=1/Rib
  Gain8 : Gain  Gain=1/Rio
  Integrator1 : Integrator  InitialCondition=Ti0
  Integrator2 : Integrator  InitialCondition=To0
  Integrator3 : Integrator  InitialCondition=Tb0
  Ta1 : InportShadow
  Tb : Outport
  Ti : Outport  Port=2
  To : Outport  Port=3
  wires:
  Integrator3/1 -> Add3/1, Add5/1, Add10/2, Add6/2, Add4/1, Tb/1
  Integrator1/1 -> Add4/2, Add6/1, Add7/1, Add8/2, Ti/1
  Integrator2/1 -> Add7/2, Add5/2, Add10/1, Add9/1, Add8/1, To/1
  Add/1 -> Gain/1
  Add1/1 -> Gain1/1
  Add2/1 -> Gain2/1
  Gain/1 -> Integrator3/1
  Gain1/1 -> Integrator1/1
  Gain2/1 -> Integrator2/1
  Pw_Bat/1 -> Add/1
  Gain4/1 -> Add/2
  Gain5/1 -> Add/3
  Gain6/1 -> Add/4
  Gain7/1 -> Add1/1
  Gain8/1 -> Add1/2
  Constant/1 -> Add2/1
  Gain13/1 -> Add2/2
  Gain14/1 -> Add2/3
  Gain11/1 -> Add2/4
  Add4/1 -> Gain4/1
  Add6/1 -> Gain7/1
  Add8/1 -> Gain13/1
  Add9/1 -> Gain14/1
  Add10/1 -> Gain11/1
  Add7/1 -> Gain8/1
  Add5/1 -> Gain6/1
  Add3/1 -> Gain5/1
  Ta/1 -> Add3/2
  Ta1/1 -> Add9/2

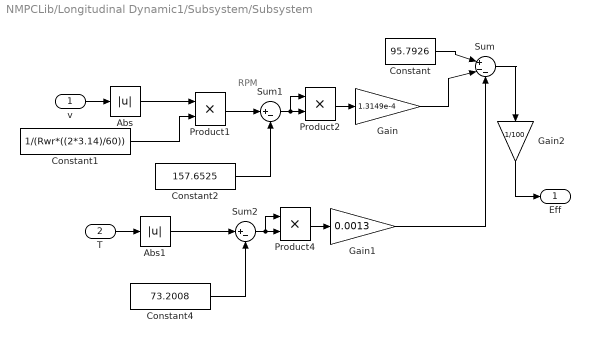
== system NMPCLib/Longitudinal Dynamic1/Subsystem/Subsystem ==
  note: RPM
  v : Inport
  T : Inport  Port=2
  Abs : Abs
  Abs1 : Abs
  Constant : Constant  Value=95.7926
  Constant1 : Constant  Value=1/(Rwr*((2*3.14)/60))
  Constant2 : Constant  Value=157.6525
  Constant4 : Constant  Value=73.2008
  Gain : Gain  Gain=1.3149e-4
  Gain1 : Gain  Gain=0.0013
  Gain2 : Gain  Gain=1/100
  Product1 : Product
  Product2 : Product
  Product4 : Product
  Sum : Sum  Inputs=|+--
  Sum1 : Sum  Inputs=|+-
  Sum2 : Sum  Inputs=|+-
  Eff : Outport
  wires:
  Abs/1 -> Product1/1
  Sum1/1 -> Product2/1, Product2/2
  Product4/1 -> Gain1/1
  Sum2/1 -> Product4/2, Product4/1
  Sum/1 -> Gain2/1
  Product2/1 -> Gain/1
  Abs1/1 -> Sum2/1
  Gain2/1 -> Eff/1
  Gain/1 -> Sum/2
  Constant4/1 -> Sum2/2
  Gain1/1 -> Sum/3
  Constant/1 -> Sum/1
  Product1/1 -> Sum1/1
  v/1 -> Abs/1
  Constant1/1 -> Product1/2
  Constant2/1 -> Sum1/2
  T/1 -> Abs1/1

== matlab function NMPCLib/Longitudinal Dynamic1/Losses Driver + Thermal/MATLAB Function ==
  data: u input; y output
function y = fcn(u)
%Calculo de la eff X=Speed, Y=Torq
Vgs       =u(1);
Rdon      =u(2);
Id        =u(3);

if Id>=0
    %%     Mosfet Conduction Losses
    Rds_on    =Rdon;
    P_drain = Rds_on*Id^2;
    
    P_d_rv = 0;    
else
    P_drain = 0;
    
    %%     Diode Conduction Losses... APLICA CUANDO LA DIRECCION DE AL CORRIENTE ES NEGATIVA
    Rd_rv =0.0033;                % CONFIRMAR autre opt = 0.0013
    Udo   =0.7;                   % CONFIRMAR
    If    =Id;
    P_d_rv=Udo*abs(If)+Rd_rv*abs(If)^2;
end

%%     Switching Losses
% Parameters
f1    = 1e3;   %[Hz]%Switching frequency (Pourteuse)
tri   = 100e-9;%[s] %DATASHEET rise time
tfi   = 30e-9; %[s] %DATASHEET fall time
Qrr   = 660e-9;%[C] %DATASHEET recovery Load

%     On current
Uplat = 5.7;      % [v]  DATASHEET Miller effect occurs and gate-source voltage is maintained at a constant level
Cgd1  = 240e-12;  % [pF] DATASHEET (Divided into two by non linearity)-> Udd/2:Udd
Cgd2  = 3300e-12; % [pF] DATASHEET (Divided into two by non linearity)-> 0    :Udd/2
Udr   = 10;       %[v]    ControlDrive Voltage
Rg    = 4.7;     %[ohm] Gate R

Igon  = (Udr-Uplat)/Rg; %V=IR
 
%     Switching ON times  (Cgd1, Cgd1)
Udd=72; %[v] Drain voltage
Tfu1=(Udd-Rdon*Igon)*Cgd1/Igon; %t=RC=V*C/I
Tfu2=(Udd-Rdon*Igon)*Cgd2/Igon; %t=RC=V*C/I
Tfu =mean([Tfu1 Tfu2]);

%     Off current
Igoff = (0-Uplat)/Rg; %V=IR

%     Switching OFF times  (Cgd1, Cgd1)
Tru1=(Udd-Rdon*Igon)*Cgd1/abs(Igoff); %t=RC=V*C/I
Tru2=(Udd-Rdon*Igon)*Cgd2/abs(Igoff); %t=RC=V*C/I
Tru =mean([Tru1 Tru2]);

%     Calculo de Energias 
Idon   = 10;        %[A] Corriente requerida  
Idoff  = 10;        %[A] Corriente requerida
Udr=Udd; % WorstCase

if Id>=0
    Wmos_on =(Udd*Idon)/2*(tri+Tfu)+Qrr*Udd;
    Wmos_off=(Udd*Idoff)/2*(Tru+tfi);
    Wd_on   =0;   
else
    Wmos_on =0;
    Wmos_off=0;
    Wd_on   =1/4*(Qrr*Udr);
end

Psw_mosf_1=1/3*(Wmos_off+Wmos_on)*f1;
Psw_d_1=1/3*(Wd_on)*f1;

Psw_mof_d_1 =Psw_mosf_1+Psw_d_1; %La potencia de perdida con corriente reverse de UN mosfet
%Psw_mof_nd_1=Psw_mosf_1;         %La potencia de perdida sin corriente reverse de UN mosfet

Pow_LosInv = P_drain+P_d_rv+Psw_mof_d_1; %Dejo positivo para que al sumar -++... suba

y = Pow_LosInv;

== matlab function NMPCLib/NMPC_N//GMRES/Solver ==
  data: dU0 input; dU output; U0 input; x0 input; TVP input; U output; Control output; TVP_f input
%% NGMRES  NGMRES NGMRES
function [dU,U,Control] = NMPCBlock(dU0,U0,x0,TVP,TVP_f)
[dU,U,Control]=NMPC(dU0,U0,x0,TVP,TVP_f);
